simulink library "libturbines"  (R2025b)
settings: Solver=ode45  StartTime=0.0  StopTime=10.0  RelTol=1e-3  EnableMultiTasking=on
undefined symbols (not defined in the file): DiscIntNeverNeededParam, dt, faultOptions, noiseFlag
libraries: simulink x57, $bdroot x3
(part 4 of 5)

== system libturbines/Floating NREL5MW faulty/Controller/Region check ==
  Torque_dem : Inport
  w_gen : Inport  Port=2
  p_dem : Inport  Port=3
  pitch command : Inport  Port=4
  Demand limitation : RelationalOperator  Operator=<=  OutDataTypeStr=boolean  InputSameDT=off
  Divide : Product  Inputs=*/
  Enable Pitch control? : Logic  Operator=OR  Inputs=3  AllPortsSameDT=off  OutDataTypeStr=boolean
  Integer Delay : Delay  DelayLength=1
  Pitch actuator active last time? : simulink/Logic and Bit Operations/Compare To Constant  relop=>  const=wt.ctrl.torq.beta  OutDataTypeStr=uint8  ZeroCross=off
  Product : Product  RndMeth=Zero
  Region 3 speed? : simulink/Logic and Bit Operations/Compare To Constant  relop=>=  const=wt.ctrl.torq.r3  OutDataTypeStr=uint8  ZeroCross=off
  Switch Torque_ref : Switch  Threshold=1  SaturateOnIntegerOverflow=off  InputSameDT=off
  Torque_ref : Outport
  Enable pitch controller : Outport  Port=2
  wires:
  Divide/1 -> Switch Torque_ref/1
  Switch Torque_ref/1 -> Torque_ref/1
  Demand limitation/1 -> Enable Pitch control?/1
  p_dem/1 -> Divide/1, Demand limitation/1
  Torque_dem/1 -> Switch Torque_ref/3, Product/1
  Product/1 -> Demand limitation/2
  Enable Pitch control?/1 -> Switch Torque_ref/2, Enable pitch controller/1
  Integer Delay/1 -> Pitch actuator active last time?/1
  Region 3 speed?/1 -> Enable Pitch control?/2
  Pitch actuator active last time?/1 -> Enable Pitch control?/3
  w_gen/1 -> Product/2, Region 3 speed?/1, Divide/2
  pitch command/1 -> Integer Delay/1

== system libturbines/Floating NREL5MW faulty/Pitch Actuator/Pitch subsystems ==
  beta_ref [deg] : Inport
  Fault type 5 : Inport  Port=2
  Demux2 : Demux  Outputs=3
  Mux1 : Mux  Inputs=3
  Pitch system B1 : StateSpace  A=wt.pitch.ssA  B=wt.pitch.ssB  C=wt.pitch.ssC  D=wt.pitch.ssD  InitialCondition=0
  Pitch system B2 : StateSpace  A=wt.pitch.ssA  B=wt.pitch.ssB  C=wt.pitch.ssC  D=wt.pitch.ssD  InitialCondition=0
  Pitch system B3 : Subsystem
  beta [deg] : Outport
  wires:
  Pitch system B3/1(beta [deg]) -> Mux1/3
  Demux2/3 -> Pitch system B3/1(beta_ref [deg])
  Fault type 5/1 -> Pitch system B3/2(fault 5)
  beta_ref [deg]/1 -> Demux2/1
  Mux1/1 -> beta [deg]/1
  Pitch system B2/1 -> Mux1/2
  Pitch system B1/1 -> Mux1/1
  Demux2/1 -> Pitch system B1/1
  Demux2/2 -> Pitch system B2/1

== system libturbines/Floating NREL5MW faulty/Sensors sampling/generator encoder ==
  w_gen_in : Inport
  Sum : Sum  Inputs=-+|
  gen Integrator : Integrator  InitialCondition=wt.gen.ini
  gen sensor time constant : Gain  Gain=1/wt.meas.gentau
  w_gen_out : Outport
  wires:
  gen Integrator/1 -> w_gen_out/1, Sum/1
  Sum/1 -> gen sensor time constant/1
  gen sensor time constant/1 -> gen Integrator/1
  w_gen_in/1 -> Sum/2

== system libturbines/Floating NREL5MW faulty/Sensors sampling/rotor encoder ==
  w_rot_in : Inport
  Sum1 : Sum  Inputs=|+-
  gen Integrator1 : Integrator  InitialCondition=wt.rotor.ini
  gen sensor time constant1 : Gain  Gain=1/wt.meas.rottau
  w_rot_out : Outport
  wires:
  w_rot_in/1 -> Sum1/1
  gen Integrator1/1 -> w_rot_out/1, Sum1/2
  Sum1/1 -> gen sensor time constant1/1
  gen sensor time constant1/1 -> gen Integrator1/1

== system libturbines/Floating NREL5MW faulty/Tower deflection /Tower1 ==
  FT [Nm] : Inport
  Demux1 : Demux  Outputs=2
  Tower : StateSpace  A=A  B=B  C=C  D=D  InitialCondition=zeros(2,1)
  vnac [m/s] : Outport  InitialOutput=0
  F_tow [N] : Outport  Port=2  InitialOutput=0
  wires:
  Demux1/2 -> F_tow [N]/1
  FT [Nm]/1 -> Tower/1
  Demux1/1 -> vnac [m/s]/1
  Tower/1 -> Demux1/1

== system libturbines/Floating IEA15MW/Controller/Pitch controller/Blade 1 controller ==
  w_gen_diff : Inport
  P_dem : Inport  Port=2
  beta_meas [deg] : Inport  Port=3
  Discrete-Time Integrator : DiscreteIntegrator  SampleTime=wt.ctrl.Ts  LimitOutput=on  UpperSaturationLimit=wt.ctrl.pitch.ulim*pi/180  LowerSaturationLimit=wt.ctrl.pitch.llim  ICPrevOutput=DiscIntNeverNeededParam  ICPrevScaledInput=DiscIntNeverNeededParam
  Gain correction : Lookup2D  RowIndex=wt.ctrl.pitch.pwr  ColumnIndex=wt.ctrl.pitch.beta  Table=wt.ctrl.pitch.gs  LookUpMeth=Interpolation-Use End Values  SaturateOnIntegerOverflow=off  InputSameDT=off
  Integral gain : Gain  Gain=(1-0.999*noiseFlag)*wt.ctrl.pitch.Igain
  Integral schedule : Product  Inputs=*/  RndMeth=Zero
  Prop schedule : Product  Inputs=*/  RndMeth=Zero
  Proportional gain : Gain  Gain=(1-0.3*noiseFlag)*wt.ctrl.pitch.Pgain
  Rate Limiter : RateLimiter  RisingSlewLimit=wt.ctrl.pitch.ratelim  FallingSlewLimit=-wt.ctrl.pitch.ratelim  SampleTimeMode=inherited  InitialCondition=wt.ctrl.pitch.ini
  Saturation : Saturate  UpperLimit=wt.ctrl.pitch.ulim  LowerLimit=0
  Sum : Sum  Inputs=++|
  To degrees : Gain  Gain=180/pi
  beta_ref [deg] : Outport
  wires:
  Integral schedule/1 -> Discrete-Time Integrator/1
  Integral gain/1 -> Integral schedule/1
  Gain correction/1 -> Prop schedule/2, Integral schedule/2
  Sum/1 -> To degrees/1
  w_gen_diff/1 -> Integral gain/1, Proportional gain/1
  To degrees/1 -> Saturation/1
  Prop schedule/1 -> Sum/1
  Saturation/1 -> Rate Limiter/1
  Discrete-Time Integrator/1 -> Sum/2
  Proportional gain/1 -> Prop schedule/1
  beta_meas [deg]/1 -> Gain correction/2
  Rate Limiter/1 -> beta_ref [deg]/1
  P_dem/1 -> Gain correction/1

== system libturbines/Floating IEA15MW faulty/Aerodynamics/Blade 1/C_P & C_T tables ==
  beta : Inport
  lambda : Inport  Port=2
  "C_P table " : Lookup2D  RowIndex=wt.cp.beta  ColumnIndex=wt.cp.tsr  Table=wt.cp.table  LookUpMeth=Interpolation-Use End Values
  C_T table : Lookup2D  RowIndex=wt.ct.beta  ColumnIndex=wt.ct.tsr  Table=wt.ct.table  LookUpMeth=Interpolation-Use End Values
  C_T : Outport
  C_P : Outport  Port=2
  wires:
  lambda/1 -> "C_P table "/2, C_T table/2
  beta/1 -> "C_P table "/1, C_T table/1
  "C_P table "/1 -> C_P/1
  C_T table/1 -> C_T/1

== system libturbines/Floating IEA15MW faulty/Aerodynamics/Blade 2/C_P & C_T tables ==
  beta : Inport
  lambda : Inport  Port=2
  "C_P table " : Lookup2D  RowIndex=wt.cp.beta  ColumnIndex=wt.cp.tsr  Table=wt.cp.table  LookUpMeth=Interpolation-Use End Values
  C_T table : Lookup2D  RowIndex=wt.ct.beta  ColumnIndex=wt.ct.tsr  Table=wt.ct.table  LookUpMeth=Interpolation-Use End Values
  C_T : Outport
  C_P : Outport  Port=2
  wires:
  lambda/1 -> "C_P table "/2, C_T table/2
  beta/1 -> "C_P table "/1, C_T table/1
  "C_P table "/1 -> C_P/1
  C_T table/1 -> C_T/1

== system libturbines/Floating IEA15MW faulty/Aerodynamics/Blade 3/C_P & C_T tables ==
  beta : Inport
  lambda : Inport  Port=2
  "C_P table " : Lookup2D  RowIndex=wt.cp.beta  ColumnIndex=wt.cp.tsr  Table=wt.cp.table  LookUpMeth=Interpolation-Use End Values
  C_T table : Lookup2D  RowIndex=wt.ct.beta  ColumnIndex=wt.ct.tsr  Table=wt.ct.table  LookUpMeth=Interpolation-Use End Values
  C_T : Outport
  C_P : Outport  Port=2
  wires:
  lambda/1 -> "C_P table "/2, C_T table/2
  beta/1 -> "C_P table "/1, C_T table/1
  "C_P table "/1 -> C_P/1
  C_T table/1 -> C_T/1

== system libturbines/Floating IEA15MW faulty/Controller/Pitch controller/Blade 1 controller ==
  w_gen_diff : Inport
  P_dem : Inport  Port=2
  beta_meas [deg] : Inport  Port=3
  Discrete-Time Integrator : DiscreteIntegrator  SampleTime=wt.ctrl.Ts  LimitOutput=on  UpperSaturationLimit=wt.ctrl.pitch.ulim*pi/180  LowerSaturationLimit=wt.ctrl.pitch.llim  ICPrevOutput=DiscIntNeverNeededParam  ICPrevScaledInput=DiscIntNeverNeededParam
  Gain correction : Lookup2D  RowIndex=wt.ctrl.pitch.pwr  ColumnIndex=wt.ctrl.pitch.beta  Table=wt.ctrl.pitch.gs  LookUpMeth=Interpolation-Use End Values  SaturateOnIntegerOverflow=off  InputSameDT=off
  Integral gain : Gain  Gain=(1-0.999*noiseFlag)*wt.ctrl.pitch.Igain
  Integral schedule : Product  Inputs=*/  RndMeth=Zero
  Prop schedule : Product  Inputs=*/  RndMeth=Zero
  Proportional gain : Gain  Gain=(1-0.3*noiseFlag)*wt.ctrl.pitch.Pgain
  Rate Limiter : RateLimiter  RisingSlewLimit=wt.ctrl.pitch.ratelim  FallingSlewLimit=-wt.ctrl.pitch.ratelim  SampleTimeMode=inherited  InitialCondition=wt.ctrl.pitch.ini
  Saturation : Saturate  UpperLimit=wt.ctrl.pitch.ulim  LowerLimit=0
  Sum : Sum  Inputs=++|
  To degrees : Gain  Gain=180/pi
  beta_ref [deg] : Outport
  wires:
  P_dem/1 -> Gain correction/1
  Rate Limiter/1 -> beta_ref [deg]/1
  beta_meas [deg]/1 -> Gain correction/2
  Proportional gain/1 -> Prop schedule/1
  Discrete-Time Integrator/1 -> Sum/2
  Saturation/1 -> Rate Limiter/1
  Prop schedule/1 -> Sum/1
  To degrees/1 -> Saturation/1
  w_gen_diff/1 -> Integral gain/1, Proportional gain/1
  Sum/1 -> To degrees/1
  Gain correction/1 -> Integral schedule/2, Prop schedule/2
  Integral gain/1 -> Integral schedule/1
  Integral schedule/1 -> Discrete-Time Integrator/1

== system libturbines/Floating IEA15MW faulty/Controller/Pitch controller/Blade 2 controller ==
  w_gen_diff : Inport
  P_dem : Inport  Port=2
  beta_meas [deg] : Inport  Port=3
  Discrete-Time Integrator : DiscreteIntegrator  SampleTime=wt.ctrl.Ts  LimitOutput=on  UpperSaturationLimit=wt.ctrl.pitch.ulim*pi/180  LowerSaturationLimit=wt.ctrl.pitch.llim  ICPrevOutput=DiscIntNeverNeededParam  ICPrevScaledInput=DiscIntNeverNeededParam
  Gain correction : Lookup2D  RowIndex=wt.ctrl.pitch.pwr  ColumnIndex=wt.ctrl.pitch.beta  Table=wt.ctrl.pitch.gs  LookUpMeth=Interpolation-Use End Values  SaturateOnIntegerOverflow=off  InputSameDT=off
  Integral gain : Gain  Gain=(1-0.999*noiseFlag)*wt.ctrl.pitch.Igain
  Integral schedule : Product  Inputs=*/  RndMeth=Zero
  Prop schedule : Product  Inputs=*/  RndMeth=Zero
  Proportional gain : Gain  Gain=(1-0.3*noiseFlag)*wt.ctrl.pitch.Pgain
  Rate Limiter : RateLimiter  RisingSlewLimit=wt.ctrl.pitch.ratelim  FallingSlewLimit=-wt.ctrl.pitch.ratelim  SampleTimeMode=inherited  InitialCondition=wt.ctrl.pitch.ini
  Saturation : Saturate  UpperLimit=wt.ctrl.pitch.ulim  LowerLimit=0
  Sum : Sum  Inputs=++|
  To degrees : Gain  Gain=180/pi
  beta_ref [deg] : Outport
  wires:
  Integral schedule/1 -> Discrete-Time Integrator/1
  Integral gain/1 -> Integral schedule/1
  Gain correction/1 -> Prop schedule/2, Integral schedule/2
  Sum/1 -> To degrees/1
  w_gen_diff/1 -> Proportional gain/1, Integral gain/1
  To degrees/1 -> Saturation/1
  Prop schedule/1 -> Sum/1
  Saturation/1 -> Rate Limiter/1
  Discrete-Time Integrator/1 -> Sum/2
  Proportional gain/1 -> Prop schedule/1
  beta_meas [deg]/1 -> Gain correction/2
  Rate Limiter/1 -> beta_ref [deg]/1
  P_dem/1 -> Gain correction/1

== system libturbines/Floating IEA15MW faulty/Controller/Pitch controller/Blade 3 controller ==
  w_gen_diff : Inport
  P_dem : Inport  Port=2
  beta_meas [deg] : Inport  Port=3
  Discrete-Time Integrator : DiscreteIntegrator  SampleTime=wt.ctrl.Ts  LimitOutput=on  UpperSaturationLimit=wt.ctrl.pitch.ulim*pi/180  LowerSaturationLimit=wt.ctrl.pitch.llim  ICPrevOutput=DiscIntNeverNeededParam  ICPrevScaledInput=DiscIntNeverNeededParam
  Gain correction : Lookup2D  RowIndex=wt.ctrl.pitch.pwr  ColumnIndex=wt.ctrl.pitch.beta  Table=wt.ctrl.pitch.gs  LookUpMeth=Interpolation-Use End Values  SaturateOnIntegerOverflow=off  InputSameDT=off
  Integral gain : Gain  Gain=(1-0.999*noiseFlag)*wt.ctrl.pitch.Igain
  Integral schedule : Product  Inputs=*/  RndMeth=Zero
  Prop schedule : Product  Inputs=*/  RndMeth=Zero
  Proportional gain : Gain  Gain=(1-0.3*noiseFlag)*wt.ctrl.pitch.Pgain
  Rate Limiter : RateLimiter  RisingSlewLimit=wt.ctrl.pitch.ratelim  FallingSlewLimit=-wt.ctrl.pitch.ratelim  SampleTimeMode=inherited  InitialCondition=wt.ctrl.pitch.ini
  Saturation : Saturate  UpperLimit=wt.ctrl.pitch.ulim  LowerLimit=0
  Sum : Sum  Inputs=++|
  To degrees : Gain  Gain=180/pi
  beta_ref [deg] : Outport
  wires:
  P_dem/1 -> Gain correction/1
  Rate Limiter/1 -> beta_ref [deg]/1
  beta_meas [deg]/1 -> Gain correction/2
  Proportional gain/1 -> Prop schedule/1
  Discrete-Time Integrator/1 -> Sum/2
  Saturation/1 -> Rate Limiter/1
  Prop schedule/1 -> Sum/1
  To degrees/1 -> Saturation/1
  w_gen_diff/1 -> Integral gain/1, Proportional gain/1
  Sum/1 -> To degrees/1
  Gain correction/1 -> Integral schedule/2, Prop schedule/2
  Integral gain/1 -> Integral schedule/1
  Integral schedule/1 -> Discrete-Time Integrator/1

== system libturbines/Floating IEA15MW faulty/Pitch Actuator/Pitch subsystems/Pitch system B3 ==
  beta_ref [deg] : Inport
  fault 5 : Inport  Port=2
  Compare To Constant : simulink/Logic and Bit Operations/Compare To Constant  relop===  const=5  OutDataTypeStr=boolean
  Constant : Constant  Value=wt.pitch.omega
  Constant1 : Constant  Value=wt.pitch.damp
  Constant2 : Constant
  Constant3 : Constant  Value=faultOptions.pitchNatFreq
  Constant4 : Constant  Value=faultOptions.pitchDamp
  Demux1 : Demux  Outputs=2
  Gain2 : Gain  Gain=2
  Integrator : Integrator
  Integrator1 : Integrator
  Product{1..3,5} (4 alike) : Product
  Signal Specification : SignalSpecification  OutDataTypeStr=double  Dimensions=1
  Square : Math  Operator=square
  Sum : Sum  Inputs=-+-
  Sum1 : Sum  Inputs=|+-
  Switch1 : Switch  Criteria=u2 ~= 0  SaturateOnIntegerOverflow=off  InputSameDT=off
  mux1 : Mux  Inputs=2
  mux2 : Mux  Inputs=2
  beta [deg] : Outport
  wires:
  Sum1/1 -> Switch1/2
  Product1/1 -> Sum/2
  Product3/1 -> Sum/1
  Constant/1 -> mux1/1
  Gain2/1 -> Product2/2
  Integrator1/1 -> Signal Specification/1, Product3/2
  Demux1/2 -> Product5/2
  Integrator/1 -> Product2/1, Integrator1/1
  Compare To Constant/1 -> Sum1/1
  Demux1/1 -> Product5/1, Square/1
  fault 5/1 -> Compare To Constant/1
  Constant2/1 -> Sum1/2
  Signal Specification/1 -> beta [deg]/1
  mux2/1 -> Switch1/3
  Sum/1 -> Integrator/1
  Square/1 -> Product3/1, Product1/2
  beta_ref [deg]/1 -> Product1/1
  Constant4/1 -> mux2/2
  mux1/1 -> Switch1/1
  Constant1/1 -> mux1/2
  Constant3/1 -> mux2/1
  Product5/1 -> Gain2/1
  Switch1/1 -> Demux1/1
  Product2/1 -> Sum/3

== system libturbines/Floating IEA3.4MW/Controller/Pitch controller/Blade 1 controller ==
  w_gen_diff : Inport
  P_dem : Inport  Port=2
  beta_meas [deg] : Inport  Port=3
  Discrete-Time Integrator : DiscreteIntegrator  SampleTime=wt.ctrl.Ts  LimitOutput=on  UpperSaturationLimit=wt.ctrl.pitch.ulim*pi/180  LowerSaturationLimit=wt.ctrl.pitch.llim  ICPrevOutput=DiscIntNeverNeededParam  ICPrevScaledInput=DiscIntNeverNeededParam
  Gain correction : Lookup2D  RowIndex=wt.ctrl.pitch.pwr  ColumnIndex=wt.ctrl.pitch.beta  Table=wt.ctrl.pitch.gs  LookUpMeth=Interpolation-Use End Values  SaturateOnIntegerOverflow=off  InputSameDT=off
  Integral gain : Gain  Gain=(1-0.999*noiseFlag)*wt.ctrl.pitch.Igain
  Integral schedule : Product  Inputs=*/  RndMeth=Zero
  Prop schedule : Product  Inputs=*/  RndMeth=Zero
  Proportional gain : Gain  Gain=(1-0.3*noiseFlag)*wt.ctrl.pitch.Pgain
  Rate Limiter : RateLimiter  RisingSlewLimit=wt.ctrl.pitch.ratelim  FallingSlewLimit=-wt.ctrl.pitch.ratelim  SampleTimeMode=inherited  InitialCondition=wt.ctrl.pitch.ini
  Saturation : Saturate  UpperLimit=wt.ctrl.pitch.ulim  LowerLimit=0
  Sum : Sum  Inputs=++|
  To degrees : Gain  Gain=180/pi
  beta_ref [deg] : Outport
  wires:
  Integral schedule/1 -> Discrete-Time Integrator/1
  Integral gain/1 -> Integral schedule/1
  Gain correction/1 -> Prop schedule/2, Integral schedule/2
  Sum/1 -> To degrees/1
  w_gen_diff/1 -> Integral gain/1, Proportional gain/1
  To degrees/1 -> Saturation/1
  Prop schedule/1 -> Sum/1
  Saturation/1 -> Rate Limiter/1
  Discrete-Time Integrator/1 -> Sum/2
  Proportional gain/1 -> Prop schedule/1
  beta_meas [deg]/1 -> Gain correction/2
  Rate Limiter/1 -> beta_ref [deg]/1
  P_dem/1 -> Gain correction/1

== system libturbines/Floating IEA3.4MW faulty/Aerodynamics/Blade 1/C_P & C_T tables ==
  beta : Inport
  lambda : Inport  Port=2
  "C_P table " : Lookup2D  RowIndex=wt.cp.beta  ColumnIndex=wt.cp.tsr  Table=wt.cp.table  LookUpMeth=Interpolation-Use End Values
  C_T table : Lookup2D  RowIndex=wt.ct.beta  ColumnIndex=wt.ct.tsr  Table=wt.ct.table  LookUpMeth=Interpolation-Use End Values
  C_T : Outport
  C_P : Outport  Port=2
  wires:
  lambda/1 -> "C_P table "/2, C_T table/2
  beta/1 -> "C_P table "/1, C_T table/1
  "C_P table "/1 -> C_P/1
  C_T table/1 -> C_T/1

== system libturbines/Floating IEA3.4MW faulty/Aerodynamics/Blade 2/C_P & C_T tables ==
  beta : Inport
  lambda : Inport  Port=2
  "C_P table " : Lookup2D  RowIndex=wt.cp.beta  ColumnIndex=wt.cp.tsr  Table=wt.cp.table  LookUpMeth=Interpolation-Use End Values
  C_T table : Lookup2D  RowIndex=wt.ct.beta  ColumnIndex=wt.ct.tsr  Table=wt.ct.table  LookUpMeth=Interpolation-Use End Values
  C_T : Outport
  C_P : Outport  Port=2
  wires:
  lambda/1 -> "C_P table "/2, C_T table/2
  beta/1 -> "C_P table "/1, C_T table/1
  "C_P table "/1 -> C_P/1
  C_T table/1 -> C_T/1

== system libturbines/Floating IEA3.4MW faulty/Aerodynamics/Blade 3/C_P & C_T tables ==
  beta : Inport
  lambda : Inport  Port=2
  "C_P table " : Lookup2D  RowIndex=wt.cp.beta  ColumnIndex=wt.cp.tsr  Table=wt.cp.table  LookUpMeth=Interpolation-Use End Values
  C_T table : Lookup2D  RowIndex=wt.ct.beta  ColumnIndex=wt.ct.tsr  Table=wt.ct.table  LookUpMeth=Interpolation-Use End Values
  C_T : Outport
  C_P : Outport  Port=2
  wires:
  lambda/1 -> "C_P table "/2, C_T table/2
  beta/1 -> "C_P table "/1, C_T table/1
  "C_P table "/1 -> C_P/1
  C_T table/1 -> C_T/1

== system libturbines/Floating IEA3.4MW faulty/Controller/Pitch controller/Blade 1 controller ==
  w_gen_diff : Inport
  P_dem : Inport  Port=2
  beta_meas [deg] : Inport  Port=3
  Discrete-Time Integrator : DiscreteIntegrator  SampleTime=wt.ctrl.Ts  LimitOutput=on  UpperSaturationLimit=wt.ctrl.pitch.ulim*pi/180  LowerSaturationLimit=wt.ctrl.pitch.llim  ICPrevOutput=DiscIntNeverNeededParam  ICPrevScaledInput=DiscIntNeverNeededParam
  Gain correction : Lookup2D  RowIndex=wt.ctrl.pitch.pwr  ColumnIndex=wt.ctrl.pitch.beta  Table=wt.ctrl.pitch.gs  LookUpMeth=Interpolation-Use End Values  SaturateOnIntegerOverflow=off  InputSameDT=off
  Integral gain : Gain  Gain=(1-0.999*noiseFlag)*wt.ctrl.pitch.Igain
  Integral schedule : Product  Inputs=*/  RndMeth=Zero
  Prop schedule : Product  Inputs=*/  RndMeth=Zero
  Proportional gain : Gain  Gain=(1-0.3*noiseFlag)*wt.ctrl.pitch.Pgain
  Rate Limiter : RateLimiter  RisingSlewLimit=wt.ctrl.pitch.ratelim  FallingSlewLimit=-wt.ctrl.pitch.ratelim  SampleTimeMode=inherited  InitialCondition=wt.ctrl.pitch.ini
  Saturation : Saturate  UpperLimit=wt.ctrl.pitch.ulim  LowerLimit=0
  Sum : Sum  Inputs=++|
  To degrees : Gain  Gain=180/pi
  beta_ref [deg] : Outport
  wires:
  P_dem/1 -> Gain correction/1
  Rate Limiter/1 -> beta_ref [deg]/1
  beta_meas [deg]/1 -> Gain correction/2
  Proportional gain/1 -> Prop schedule/1
  Discrete-Time Integrator/1 -> Sum/2
  Saturation/1 -> Rate Limiter/1
  Prop schedule/1 -> Sum/1
  To degrees/1 -> Saturation/1
  w_gen_diff/1 -> Integral gain/1, Proportional gain/1
  Sum/1 -> To degrees/1
  Gain correction/1 -> Integral schedule/2, Prop schedule/2
  Integral gain/1 -> Integral schedule/1
  Integral schedule/1 -> Discrete-Time Integrator/1

== system libturbines/Floating IEA3.4MW faulty/Controller/Pitch controller/Blade 2 controller ==
  w_gen_diff : Inport
  P_dem : Inport  Port=2
  beta_meas [deg] : Inport  Port=3
  Discrete-Time Integrator : DiscreteIntegrator  SampleTime=wt.ctrl.Ts  LimitOutput=on  UpperSaturationLimit=wt.ctrl.pitch.ulim*pi/180  LowerSaturationLimit=wt.ctrl.pitch.llim  ICPrevOutput=DiscIntNeverNeededParam  ICPrevScaledInput=DiscIntNeverNeededParam
  Gain correction : Lookup2D  RowIndex=wt.ctrl.pitch.pwr  ColumnIndex=wt.ctrl.pitch.beta  Table=wt.ctrl.pitch.gs  LookUpMeth=Interpolation-Use End Values  SaturateOnIntegerOverflow=off  InputSameDT=off
  Integral gain : Gain  Gain=(1-0.999*noiseFlag)*wt.ctrl.pitch.Igain
  Integral schedule : Product  Inputs=*/  RndMeth=Zero
  Prop schedule : Product  Inputs=*/  RndMeth=Zero
  Proportional gain : Gain  Gain=(1-0.3*noiseFlag)*wt.ctrl.pitch.Pgain
  Rate Limiter : RateLimiter  RisingSlewLimit=wt.ctrl.pitch.ratelim  FallingSlewLimit=-wt.ctrl.pitch.ratelim  SampleTimeMode=inherited  InitialCondition=wt.ctrl.pitch.ini
  Saturation : Saturate  UpperLimit=wt.ctrl.pitch.ulim  LowerLimit=0
  Sum : Sum  Inputs=++|
  To degrees : Gain  Gain=180/pi
  beta_ref [deg] : Outport
  wires:
  Integral schedule/1 -> Discrete-Time Integrator/1
  Integral gain/1 -> Integral schedule/1
  Gain correction/1 -> Prop schedule/2, Integral schedule/2
  Sum/1 -> To degrees/1
  w_gen_diff/1 -> Proportional gain/1, Integral gain/1
  To degrees/1 -> Saturation/1
  Prop schedule/1 -> Sum/1
  Saturation/1 -> Rate Limiter/1
  Discrete-Time Integrator/1 -> Sum/2
  Proportional gain/1 -> Prop schedule/1
  beta_meas [deg]/1 -> Gain correction/2
  Rate Limiter/1 -> beta_ref [deg]/1
  P_dem/1 -> Gain correction/1

== system libturbines/Floating IEA3.4MW faulty/Controller/Pitch controller/Blade 3 controller ==
  w_gen_diff : Inport
  P_dem : Inport  Port=2
  beta_meas [deg] : Inport  Port=3
  Discrete-Time Integrator : DiscreteIntegrator  SampleTime=wt.ctrl.Ts  LimitOutput=on  UpperSaturationLimit=wt.ctrl.pitch.ulim*pi/180  LowerSaturationLimit=wt.ctrl.pitch.llim  ICPrevOutput=DiscIntNeverNeededParam  ICPrevScaledInput=DiscIntNeverNeededParam
  Gain correction : Lookup2D  RowIndex=wt.ctrl.pitch.pwr  ColumnIndex=wt.ctrl.pitch.beta  Table=wt.ctrl.pitch.gs  LookUpMeth=Interpolation-Use End Values  SaturateOnIntegerOverflow=off  InputSameDT=off
  Integral gain : Gain  Gain=(1-0.999*noiseFlag)*wt.ctrl.pitch.Igain
  Integral schedule : Product  Inputs=*/  RndMeth=Zero
  Prop schedule : Product  Inputs=*/  RndMeth=Zero
  Proportional gain : Gain  Gain=(1-0.3*noiseFlag)*wt.ctrl.pitch.Pgain
  Rate Limiter : RateLimiter  RisingSlewLimit=wt.ctrl.pitch.ratelim  FallingSlewLimit=-wt.ctrl.pitch.ratelim  SampleTimeMode=inherited  InitialCondition=wt.ctrl.pitch.ini
  Saturation : Saturate  UpperLimit=wt.ctrl.pitch.ulim  LowerLimit=0
  Sum : Sum  Inputs=++|
  To degrees : Gain  Gain=180/pi
  beta_ref [deg] : Outport
  wires:
  P_dem/1 -> Gain correction/1
  Rate Limiter/1 -> beta_ref [deg]/1
  beta_meas [deg]/1 -> Gain correction/2
  Proportional gain/1 -> Prop schedule/1
  Discrete-Time Integrator/1 -> Sum/2
  Saturation/1 -> Rate Limiter/1
  Prop schedule/1 -> Sum/1
  To degrees/1 -> Saturation/1
  w_gen_diff/1 -> Integral gain/1, Proportional gain/1
  Sum/1 -> To degrees/1
  Gain correction/1 -> Integral schedule/2, Prop schedule/2
  Integral gain/1 -> Integral schedule/1
  Integral schedule/1 -> Discrete-Time Integrator/1

== system libturbines/Floating IEA3.4MW faulty/Pitch Actuator/Pitch subsystems/Pitch system B3 ==
  beta_ref [deg] : Inport
  fault 5 : Inport  Port=2
  Compare To Constant : simulink/Logic and Bit Operations/Compare To Constant  relop===  const=5  OutDataTypeStr=boolean
  Constant : Constant  Value=wt.pitch.omega
  Constant1 : Constant  Value=wt.pitch.damp
  Constant2 : Constant
  Constant3 : Constant  Value=faultOptions.pitchNatFreq
  Constant4 : Constant  Value=faultOptions.pitchDamp
  Demux1 : Demux  Outputs=2
  Gain2 : Gain  Gain=2
  Integrator : Integrator
  Integrator1 : Integrator
  Product{1..3,5} (4 alike) : Product
  Signal Specification : SignalSpecification  OutDataTypeStr=double  Dimensions=1
  Square : Math  Operator=square
  Sum : Sum  Inputs=-+-
  Sum1 : Sum  Inputs=|+-
  Switch1 : Switch  Criteria=u2 ~= 0  SaturateOnIntegerOverflow=off  InputSameDT=off
  mux1 : Mux  Inputs=2
  mux2 : Mux  Inputs=2
  beta [deg] : Outport
  wires:
  Sum1/1 -> Switch1/2
  Product1/1 -> Sum/2
  Product3/1 -> Sum/1
  Constant/1 -> mux1/1
  Gain2/1 -> Product2/2
  Integrator1/1 -> Signal Specification/1, Product3/2
  Demux1/2 -> Product5/2
  Integrator/1 -> Product2/1, Integrator1/1
  Compare To Constant/1 -> Sum1/1
  Demux1/1 -> Product5/1, Square/1
  fault 5/1 -> Compare To Constant/1
  Constant2/1 -> Sum1/2
  Signal Specification/1 -> beta [deg]/1
  mux2/1 -> Switch1/3
  Sum/1 -> Integrator/1
  Square/1 -> Product3/1, Product1/2
  beta_ref [deg]/1 -> Product1/1
  Constant4/1 -> mux2/2
  mux1/1 -> Switch1/1
  Constant1/1 -> mux1/2
  Constant3/1 -> mux2/1
  Product5/1 -> Gain2/1
  Switch1/1 -> Demux1/1
  Product2/1 -> Sum/3

== system libturbines/Floating NREL5MW/Controller/Pitch controller/Blade 1 controller ==
  w_gen_diff : Inport
  P_dem : Inport  Port=2
  beta_meas [deg] : Inport  Port=3
  Discrete-Time Integrator : DiscreteIntegrator  SampleTime=wt.ctrl.Ts  LimitOutput=on  UpperSaturationLimit=wt.ctrl.pitch.ulim*pi/180  LowerSaturationLimit=wt.ctrl.pitch.llim  ICPrevOutput=DiscIntNeverNeededParam  ICPrevScaledInput=DiscIntNeverNeededParam
  Gain correction : Lookup2D  RowIndex=wt.ctrl.pitch.pwr  ColumnIndex=wt.ctrl.pitch.beta  Table=wt.ctrl.pitch.gs  LookUpMeth=Interpolation-Use End Values  SaturateOnIntegerOverflow=off  InputSameDT=off
  Integral gain : Gain  Gain=(1-0.999*noiseFlag)*wt.ctrl.pitch.Igain
  Integral schedule : Product  Inputs=*/  RndMeth=Zero
  Prop schedule : Product  Inputs=*/  RndMeth=Zero
  Proportional gain : Gain  Gain=(1-0.3*noiseFlag)*wt.ctrl.pitch.Pgain
  Rate Limiter : RateLimiter  RisingSlewLimit=wt.ctrl.pitch.ratelim  FallingSlewLimit=-wt.ctrl.pitch.ratelim  SampleTimeMode=inherited  InitialCondition=wt.ctrl.pitch.ini
  Saturation : Saturate  UpperLimit=wt.ctrl.pitch.ulim  LowerLimit=0
  Sum : Sum  Inputs=++|
  To degrees : Gain  Gain=180/pi
  beta_ref [deg] : Outport
  wires:
  P_dem/1 -> Gain correction/1
  Rate Limiter/1 -> beta_ref [deg]/1
  beta_meas [deg]/1 -> Gain correction/2
  Proportional gain/1 -> Prop schedule/1
  Discrete-Time Integrator/1 -> Sum/2
  Saturation/1 -> Rate Limiter/1
  Prop schedule/1 -> Sum/1
  To degrees/1 -> Saturation/1
  w_gen_diff/1 -> Proportional gain/1, Integral gain/1
  Sum/1 -> To degrees/1
  Gain correction/1 -> Integral schedule/2, Prop schedule/2
  Integral gain/1 -> Integral schedule/1
  Integral schedule/1 -> Discrete-Time Integrator/1

== system libturbines/Floating NREL5MW faulty/Aerodynamics/Blade 1/C_P & C_T tables ==
  beta : Inport
  lambda : Inport  Port=2
  "C_P table " : Lookup2D  RowIndex=wt.cp.beta  ColumnIndex=wt.cp.tsr  Table=wt.cp.table  LookUpMeth=Interpolation-Use End Values
  C_T table : Lookup2D  RowIndex=wt.ct.beta  ColumnIndex=wt.ct.tsr  Table=wt.ct.table  LookUpMeth=Interpolation-Use End Values
  C_T : Outport
  C_P : Outport  Port=2
  wires:
  C_T table/1 -> C_T/1
  "C_P table "/1 -> C_P/1
  beta/1 -> C_T table/1, "C_P table "/1
  lambda/1 -> C_T table/2, "C_P table "/2

== system libturbines/Floating NREL5MW faulty/Aerodynamics/Blade 2/C_P & C_T tables ==
  beta : Inport
  lambda : Inport  Port=2
  "C_P table " : Lookup2D  RowIndex=wt.cp.beta  ColumnIndex=wt.cp.tsr  Table=wt.cp.table  LookUpMeth=Interpolation-Use End Values
  C_T table : Lookup2D  RowIndex=wt.ct.beta  ColumnIndex=wt.ct.tsr  Table=wt.ct.table  LookUpMeth=Interpolation-Use End Values
  C_T : Outport
  C_P : Outport  Port=2
  wires:
  C_T table/1 -> C_T/1
  "C_P table "/1 -> C_P/1
  beta/1 -> C_T table/1, "C_P table "/1
  lambda/1 -> C_T table/2, "C_P table "/2

== system libturbines/Floating NREL5MW faulty/Aerodynamics/Blade 3/C_P & C_T tables ==
  beta : Inport
  lambda : Inport  Port=2
  "C_P table " : Lookup2D  RowIndex=wt.cp.beta  ColumnIndex=wt.cp.tsr  Table=wt.cp.table  LookUpMeth=Interpolation-Use End Values
  C_T table : Lookup2D  RowIndex=wt.ct.beta  ColumnIndex=wt.ct.tsr  Table=wt.ct.table  LookUpMeth=Interpolation-Use End Values
  C_T : Outport
  C_P : Outport  Port=2
  wires:
  C_T table/1 -> C_T/1
  "C_P table "/1 -> C_P/1
  beta/1 -> C_T table/1, "C_P table "/1
  lambda/1 -> C_T table/2, "C_P table "/2

== system libturbines/Floating NREL5MW faulty/Controller/Pitch controller/Blade 1 controller ==
  w_gen_diff : Inport
  P_dem : Inport  Port=2
  beta_meas [deg] : Inport  Port=3
  Discrete-Time Integrator : DiscreteIntegrator  SampleTime=wt.ctrl.Ts  LimitOutput=on  UpperSaturationLimit=wt.ctrl.pitch.ulim*pi/180  LowerSaturationLimit=wt.ctrl.pitch.llim  ICPrevOutput=DiscIntNeverNeededParam  ICPrevScaledInput=DiscIntNeverNeededParam
  Gain correction : Lookup2D  RowIndex=wt.ctrl.pitch.pwr  ColumnIndex=wt.ctrl.pitch.beta  Table=wt.ctrl.pitch.gs  LookUpMeth=Interpolation-Use End Values  SaturateOnIntegerOverflow=off  InputSameDT=off
  Integral gain : Gain  Gain=(1-0.999*noiseFlag)*wt.ctrl.pitch.Igain
  Integral schedule : Product  Inputs=*/  RndMeth=Zero
  Prop schedule : Product  Inputs=*/  RndMeth=Zero
  Proportional gain : Gain  Gain=(1-0.3*noiseFlag)*wt.ctrl.pitch.Pgain
  Rate Limiter : RateLimiter  RisingSlewLimit=wt.ctrl.pitch.ratelim  FallingSlewLimit=-wt.ctrl.pitch.ratelim  SampleTimeMode=inherited  InitialCondition=wt.ctrl.pitch.ini
  Saturation : Saturate  UpperLimit=wt.ctrl.pitch.ulim  LowerLimit=0
  Sum : Sum  Inputs=++|
  To degrees : Gain  Gain=180/pi
  beta_ref [deg] : Outport
  wires:
  Integral schedule/1 -> Discrete-Time Integrator/1
  Integral gain/1 -> Integral schedule/1
  Gain correction/1 -> Prop schedule/2, Integral schedule/2
  Sum/1 -> To degrees/1
  w_gen_diff/1 -> Proportional gain/1, Integral gain/1
  To degrees/1 -> Saturation/1
  Prop schedule/1 -> Sum/1
  Saturation/1 -> Rate Limiter/1
  Discrete-Time Integrator/1 -> Sum/2
  Proportional gain/1 -> Prop schedule/1
  beta_meas [deg]/1 -> Gain correction/2
  Rate Limiter/1 -> beta_ref [deg]/1
  P_dem/1 -> Gain correction/1

== system libturbines/Floating NREL5MW faulty/Controller/Pitch controller/Blade 2 controller ==
  w_gen_diff : Inport
  P_dem : Inport  Port=2
  beta_meas [deg] : Inport  Port=3
  Discrete-Time Integrator : DiscreteIntegrator  SampleTime=wt.ctrl.Ts  LimitOutput=on  UpperSaturationLimit=wt.ctrl.pitch.ulim*pi/180  LowerSaturationLimit=wt.ctrl.pitch.llim  ICPrevOutput=DiscIntNeverNeededParam  ICPrevScaledInput=DiscIntNeverNeededParam
  Gain correction : Lookup2D  RowIndex=wt.ctrl.pitch.pwr  ColumnIndex=wt.ctrl.pitch.beta  Table=wt.ctrl.pitch.gs  LookUpMeth=Interpolation-Use End Values  SaturateOnIntegerOverflow=off  InputSameDT=off
  Integral gain : Gain  Gain=(1-0.999*noiseFlag)*wt.ctrl.pitch.Igain
  Integral schedule : Product  Inputs=*/  RndMeth=Zero
  Prop schedule : Product  Inputs=*/  RndMeth=Zero
  Proportional gain : Gain  Gain=(1-0.3*noiseFlag)*wt.ctrl.pitch.Pgain
  Rate Limiter : RateLimiter  RisingSlewLimit=wt.ctrl.pitch.ratelim  FallingSlewLimit=-wt.ctrl.pitch.ratelim  SampleTimeMode=inherited  InitialCondition=wt.ctrl.pitch.ini
  Saturation : Saturate  UpperLimit=wt.ctrl.pitch.ulim  LowerLimit=0
  Sum : Sum  Inputs=++|
  To degrees : Gain  Gain=180/pi
  beta_ref [deg] : Outport
  wires:
  P_dem/1 -> Gain correction/1
  Rate Limiter/1 -> beta_ref [deg]/1
  beta_meas [deg]/1 -> Gain correction/2
  Proportional gain/1 -> Prop schedule/1
  Discrete-Time Integrator/1 -> Sum/2
  Saturation/1 -> Rate Limiter/1
  Prop schedule/1 -> Sum/1
  To degrees/1 -> Saturation/1
  w_gen_diff/1 -> Integral gain/1, Proportional gain/1
  Sum/1 -> To degrees/1
  Gain correction/1 -> Integral schedule/2, Prop schedule/2
  Integral gain/1 -> Integral schedule/1
  Integral schedule/1 -> Discrete-Time Integrator/1

== system libturbines/Floating NREL5MW faulty/Controller/Pitch controller/Blade 3 controller ==
  w_gen_diff : Inport
  P_dem : Inport  Port=2
  beta_meas [deg] : Inport  Port=3
  Discrete-Time Integrator : DiscreteIntegrator  SampleTime=wt.ctrl.Ts  LimitOutput=on  UpperSaturationLimit=wt.ctrl.pitch.ulim*pi/180  LowerSaturationLimit=wt.ctrl.pitch.llim  ICPrevOutput=DiscIntNeverNeededParam  ICPrevScaledInput=DiscIntNeverNeededParam
  Gain correction : Lookup2D  RowIndex=wt.ctrl.pitch.pwr  ColumnIndex=wt.ctrl.pitch.beta  Table=wt.ctrl.pitch.gs  LookUpMeth=Interpolation-Use End Values  SaturateOnIntegerOverflow=off  InputSameDT=off
  Integral gain : Gain  Gain=(1-0.999*noiseFlag)*wt.ctrl.pitch.Igain
  Integral schedule : Product  Inputs=*/  RndMeth=Zero
  Prop schedule : Product  Inputs=*/  RndMeth=Zero
  Proportional gain : Gain  Gain=(1-0.3*noiseFlag)*wt.ctrl.pitch.Pgain
  Rate Limiter : RateLimiter  RisingSlewLimit=wt.ctrl.pitch.ratelim  FallingSlewLimit=-wt.ctrl.pitch.ratelim  SampleTimeMode=inherited  InitialCondition=wt.ctrl.pitch.ini
  Saturation : Saturate  UpperLimit=wt.ctrl.pitch.ulim  LowerLimit=0
  Sum : Sum  Inputs=++|
  To degrees : Gain  Gain=180/pi
  beta_ref [deg] : Outport
  wires:
  Integral schedule/1 -> Discrete-Time Integrator/1
  Integral gain/1 -> Integral schedule/1
  Gain correction/1 -> Prop schedule/2, Integral schedule/2
  Sum/1 -> To degrees/1
  w_gen_diff/1 -> Proportional gain/1, Integral gain/1
  To degrees/1 -> Saturation/1
  Prop schedule/1 -> Sum/1
  Saturation/1 -> Rate Limiter/1
  Discrete-Time Integrator/1 -> Sum/2
  Proportional gain/1 -> Prop schedule/1
  beta_meas [deg]/1 -> Gain correction/2
  Rate Limiter/1 -> beta_ref [deg]/1
  P_dem/1 -> Gain correction/1

== system libturbines/Floating NREL5MW faulty/Pitch Actuator/Pitch subsystems/Pitch system B3 ==
  beta_ref [deg] : Inport
  fault 5 : Inport  Port=2
  Compare To Constant : simulink/Logic and Bit Operations/Compare To Constant  relop===  const=5  OutDataTypeStr=boolean
  Constant : Constant  Value=wt.pitch.omega
  Constant1 : Constant  Value=wt.pitch.damp
  Constant2 : Constant
  Constant3 : Constant  Value=faultOptions.pitchNatFreq
  Constant4 : Constant  Value=faultOptions.pitchDamp
  Demux1 : Demux  Outputs=2
  Gain2 : Gain  Gain=2
  Integrator : Integrator
  Integrator1 : Integrator
  Product{1..3,5} (4 alike) : Product
  Signal Specification : SignalSpecification  OutDataTypeStr=double  Dimensions=1
  Square : Math  Operator=square
  Sum : Sum  Inputs=-+-
  Sum1 : Sum  Inputs=|+-
  Switch1 : Switch  Criteria=u2 ~= 0  SaturateOnIntegerOverflow=off  InputSameDT=off
  mux1 : Mux  Inputs=2
  mux2 : Mux  Inputs=2
  beta [deg] : Outport
  wires:
  Sum/1 -> Integrator/1
  fault 5/1 -> Compare To Constant/1
  Signal Specification/1 -> beta [deg]/1
  mux2/1 -> Switch1/3
  Constant1/1 -> mux1/2
  mux1/1 -> Switch1/1
  Product5/1 -> Gain2/1
  Product2/1 -> Sum/3
  Demux1/1 -> Product5/1, Square/1
  Constant2/1 -> Sum1/2
  Integrator/1 -> Product2/1, Integrator1/1
  Demux1/2 -> Product5/2
  Integrator1/1 -> Signal Specification/1, Product3/2
  Gain2/1 -> Product2/2
  Switch1/1 -> Demux1/1
  Constant3/1 -> mux2/1
  Constant/1 -> mux1/1
  Product3/1 -> Sum/1
  Product1/1 -> Sum/2
  Square/1 -> Product3/1, Product1/2
  Constant4/1 -> mux2/2
  Sum1/1 -> Switch1/2
  Compare To Constant/1 -> Sum1/1
  beta_ref [deg]/1 -> Product1/1

== matlab function libturbines/Floating NREL5MW faulty/Sensors sampling/Generator speed sensor fault ==
  settings: updateMethod=DISCRETE
  data: w_gen_real input; w_gen_prev input; GenSenFault input; drift_aux_in input; w_gen_meas output; faultOptions parameter; drift_aux_out output
function [w_gen_meas,drift_aux_out] = fcn(w_gen_real,w_gen_prev,GenSenFault,drift_aux_in,faultOptions)
%%%%%%%%%%%%%%%%%%%%%%%%%%%%%%%%%%%%%%%%%%%%%%%%%%%%%%%%%%%%%%%%%%%%%%%%%
% Generator speed sensor fault function
% Inputs:
%   - w_gen_real:   Real generator speed [rad/s]
%   - w_gen_prev:   Previous generator speed (measured) [rad/s]
%   - fault_type:   Desired fault type:
%                     0 - no fault
%                     1 - stuck at a fixed value
%                     2 - constant offset fault
%                     3 - drifting fault
%                     4 - constant gain fault
%                     5 - loss of precision
% Outputs:
%   - w_gen_meas:   Measured generator speed [rad/s] after the effect of the fault
%
%
% Author: Yerai Peña-Sanchez
%%%%%%%%%%%%%%%%%%%%%%%%%%%%%%%%%%%%%%%%%%%%%%%%%%%%%%%%%%%%%%%%%%%%%%%%

y_t = w_gen_real;  % Without any fault
switch floor(GenSenFault)
    case 1  % Stuck at a fixed value
        y_t = w_gen_prev;
    case 2  % Constant offset value
        y_t = w_gen_real-faultOptions.GenSenOffset;
    case 3  % Drifting value
        drift_aux_in = drift_aux_in + 1;
        y_t = w_gen_real + drift_aux_in*faultOptions.GenSenDriftSlope;
    case 4  % Constant gain value
        y_t = w_gen_real*faultOptions.GenSenGain;
    case 5  % Loss of precision of the sensor
        y_t = w_gen_real+w_gen_real*(2*rand-1)*faultOptions.GenSenPrecision;
end

if floor(GenSenFault) ~= 3
    drift_aux_out = 0;
else
    drift_aux_out = drift_aux_in;
end
w_gen_meas = y_t;

== matlab function libturbines/Floating IEA15MW faulty/Sensors sampling/Generator power sensor fault ==
  settings: updateMethod=DISCRETE
  data: p_gen_real input; p_gen_prev input; GenPSenFault input; drift_aux_in input; p_gen_meas output; faultOptions parameter; drift_aux_out output
function [p_gen_meas,drift_aux_out] = fcn(p_gen_real,p_gen_prev,GenPSenFault,drift_aux_in,faultOptions)
%%%%%%%%%%%%%%%%%%%%%%%%%%%%%%%%%%%%%%%%%%%%%%%%%%%%%%%%%%%%%%%%%%%%%%%%%
% Generator power sensor fault function
% Inputs:
%   - p_gen_real:   Real generator power [W]
%   - p_gen_prev:   Previous generator power (measured) [W]
%   - fault_type:   Desired fault type:
%                     0 - no fault
%                     1 - stuck at a fixed value
%                     2 - constant offset fault
%                     3 - drifting fault
%                     4 - constant gain fault
%                     5 - loss of precision
% Outputs:
%   - p_gen_meas:   Measured generator power [W] after the effect of the fault
%
%
% Author: Yerai Peña-Sanchez
%%%%%%%%%%%%%%%%%%%%%%%%%%%%%%%%%%%%%%%%%%%%%%%%%%%%%%%%%%%%%%%%%%%%%%%%

y_t = p_gen_real;  % Without any fault
switch floor(GenPSenFault)
    case 1  % Stuck at a fixed value
        y_t = p_gen_prev;
    case 2  % Constant offset value
        y_t = p_gen_real-faultOptions.GenPSenOffset;
    case 3  % Drifting value
        drift_aux_in = drift_aux_in + 1;
        y_t = p_gen_real + drift_aux_in*faultOptions.GenPSenDriftSlope;
    case 4  % Constant gain value
        y_t = p_gen_real*faultOptions.GenPSenGain;
    case 5  % Loss of precision of the sensor
        y_t = p_gen_real+p_gen_real*(2*rand-1)*faultOptions.GenPSenPrecision;
end

if floor(GenPSenFault) ~= 3
    drift_aux_out = 0;
else
    drift_aux_out = drift_aux_in;
end
p_gen_meas = y_t;

== matlab function libturbines/Floating NREL5MW faulty/Sensors sampling/Rotor speed sensor fault ==
  settings: updateMethod=DISCRETE
  data: w_rot_real input; w_rot_prev input; RotSenFault input; drift_aux_in input; w_rot_meas output; faultOptions parameter; drift_aux_out output
function [w_rot_meas,drift_aux_out] = fcn(w_rot_real,w_rot_prev,RotSenFault,drift_aux_in,faultOptions)
%%%%%%%%%%%%%%%%%%%%%%%%%%%%%%%%%%%%%%%%%%%%%%%%%%%%%%%%%%%%%%%%%%%%%%%%%
% Rotor speed sensor fault function
% Inputs:
%   - w_gen_real:   Real rotor speed [rad/s]
%   - w_gen_prev:   Previous generator speed (measured) [rad/s]
%   - fault_type:   Desired fault type:
%                     0 - no fault
%                     1 - stuck at a fixed value
%                     2 - constant offset fault
%                     3 - drifting fault
%                     4 - constant gain fault
%                     5 - loss of precision
% Outputs:
%   - w_rot_meas:   Measured rotor speed [rad/s] after the effect of the fault
%
%
% Author: Yerai Peña-Sanchez
%%%%%%%%%%%%%%%%%%%%%%%%%%%%%%%%%%%%%%%%%%%%%%%%%%%%%%%%%%%%%%%%%%%%%%%%

y_t = w_rot_real;  % Without any fault
switch floor(RotSenFault)
    case 1  % Stuck at a fixed value
        y_t = w_rot_prev;
    case 2  % Constant offset value
        y_t = w_rot_real-faultOptions.RotSenOffset;
    case 3  % Drifting value
        drift_aux_in = drift_aux_in + 1;
        y_t = w_rot_real + drift_aux_in*faultOptions.RotSenDriftSlope;
    case 4  % Constant gain value
        y_t = w_rot_real*faultOptions.RotSenGain;
    case 5  % Loss of precision of the sensor
        y_t = w_rot_real+w_rot_real*(2*rand-1)*faultOptions.RotSenPrecision;
end

if floor(RotSenFault) ~= 3
    drift_aux_out = 0;
else
    drift_aux_out = drift_aux_in;
end
w_rot_meas = y_t;

== matlab function libturbines/Floating NREL5MW faulty/Sensors sampling/Generator power sensor fault ==
  settings: updateMethod=DISCRETE
  data: p_gen_real input; p_gen_prev input; GenPSenFault input; drift_aux_in input; p_gen_meas output; faultOptions parameter; drift_aux_out output
function [p_gen_meas,drift_aux_out] = fcn(p_gen_real,p_gen_prev,GenPSenFault,drift_aux_in,faultOptions)
%%%%%%%%%%%%%%%%%%%%%%%%%%%%%%%%%%%%%%%%%%%%%%%%%%%%%%%%%%%%%%%%%%%%%%%%%
% Generator power sensor fault function
% Inputs:
%   - p_gen_real:   Real generator power [W]
%   - p_gen_prev:   Previous generator power (measured) [W]
%   - fault_type:   Desired fault type:
%                     0 - no fault
%                     1 - stuck at a fixed value
%                     2 - constant offset fault
%                     3 - drifting fault
%                     4 - constant gain fault
%                     5 - loss of precision
% Outputs:
%   - p_gen_meas:   Measured generator power [W] after the effect of the fault
%
%
% Author: Yerai Peña-Sanchez
%%%%%%%%%%%%%%%%%%%%%%%%%%%%%%%%%%%%%%%%%%%%%%%%%%%%%%%%%%%%%%%%%%%%%%%%

y_t = p_gen_real;  % Without any fault
switch floor(GenPSenFault)
    case 1  % Stuck at a fixed value
        y_t = p_gen_prev;
    case 2  % Constant offset value
        y_t = p_gen_real-faultOptions.GenPSenOffset;
    case 3  % Drifting value
        drift_aux_in = drift_aux_in + 1;
        y_t = p_gen_real + drift_aux_in*faultOptions.GenPSenDriftSlope;
    case 4  % Constant gain value
        y_t = p_gen_real*faultOptions.GenPSenGain;
    case 5  % Loss of precision of the sensor
        y_t = p_gen_real+p_gen_real*(2*rand-1)*faultOptions.GenPSenPrecision;
end

if floor(GenPSenFault) ~= 3
    drift_aux_out = 0;
else
    drift_aux_out = drift_aux_in;
end
p_gen_meas = y_t;

== matlab function libturbines/Floating IEA15MW faulty/Sensors sampling/Generator speed sensor fault ==
  settings: updateMethod=DISCRETE
  data: w_gen_real input; w_gen_prev input; GenSenFault input; drift_aux_in input; w_gen_meas output; faultOptions parameter; drift_aux_out output
function [w_gen_meas,drift_aux_out] = fcn(w_gen_real,w_gen_prev,GenSenFault,drift_aux_in,faultOptions)
%%%%%%%%%%%%%%%%%%%%%%%%%%%%%%%%%%%%%%%%%%%%%%%%%%%%%%%%%%%%%%%%%%%%%%%%%
% Generator speed sensor fault function
% Inputs:
%   - w_gen_real:   Real generator speed [rad/s]
%   - w_gen_prev:   Previous generator speed (measured) [rad/s]
%   - fault_type:   Desired fault type:
%                     0 - no fault
%                     1 - stuck at a fixed value
%                     2 - constant offset fault
%                     3 - drifting fault
%                     4 - constant gain fault
%                     5 - loss of precision
% Outputs:
%   - w_gen_meas:   Measured generator speed [rad/s] after the effect of the fault
%
%
% Author: Yerai Peña-Sanchez
%%%%%%%%%%%%%%%%%%%%%%%%%%%%%%%%%%%%%%%%%%%%%%%%%%%%%%%%%%%%%%%%%%%%%%%%

y_t = w_gen_real;  % Without any fault
switch floor(GenSenFault)
    case 1  % Stuck at a fixed value
        y_t = w_gen_prev;
    case 2  % Constant offset value
        y_t = w_gen_real-faultOptions.GenSenOffset;
    case 3  % Drifting value
        drift_aux_in = drift_aux_in + 1;
        y_t = w_gen_real + drift_aux_in*faultOptions.GenSenDriftSlope;
    case 4  % Constant gain value
        y_t = w_gen_real*faultOptions.GenSenGain;
    case 5  % Loss of precision of the sensor
        y_t = w_gen_real+w_gen_real*(2*rand-1)*faultOptions.GenSenPrecision;
end

if floor(GenSenFault) ~= 3
    drift_aux_out = 0;
else
    drift_aux_out = drift_aux_in;
end
w_gen_meas = y_t;

== matlab function libturbines/Floating IEA15MW faulty/Sensors sampling/Pitch sensor fault ==
  settings: updateMethod=DISCRETE
  data: beta_real input; beta_prev input; PitchSenFault input; drift_aux_in input; beta_meas output; faultOptions parameter; drift_aux_out output
function [beta_meas,drift_aux_out] = fcn(beta_real,beta_prev,PitchSenFault,drift_aux_in,faultOptions)
%%%%%%%%%%%%%%%%%%%%%%%%%%%%%%%%%%%%%%%%%%%%%%%%%%%%%%%%%%%%%%%%%%%%%%%%%
% Pitch sensor fault function
% Inputs:
%   - beta_real:    Real pitch angle [deg] of the actuator
%   - beta_prev:    Previous pitch angle (measured) [deg]
%   - fault_type:   Desired fault type:
%                     0 - no fault
%                     1 - stuck at a fixed value
%                     2 - constant offset fault
%                     3 - drifting fault
%                     4 - constant gain fault
%                     5 - loss of precision
% Outputs:
%   - beta_meas:    Measured pitch angle [deg] after the effect of the fault
%
%
% Author: Yerai Peña-Sanchez
%%%%%%%%%%%%%%%%%%%%%%%%%%%%%%%%%%%%%%%%%%%%%%%%%%%%%%%%%%%%%%%%%%%%%%%%

y_t = beta_real;  % Without any fault
switch floor(PitchSenFault)
    case 1  % Stuck at a fixed value
        y_t(3) = beta_prev(3);
    case 2  % Constant offset value
        y_t(3) = beta_real(3)-faultOptions.PitchSenOffset;
    case 3  % Drifting value
        drift_aux_in = drift_aux_in + 1;
        y_t(3) = beta_real(3) + drift_aux_in*faultOptions.PitchSenDriftSlope;
    case 4  % Constant gain value
        y_t(3) = beta_real(3)*faultOptions.PitchSenGain;
    case 5  % Loss of precision of the sensor
        y_t(3) = beta_real(3)+beta_real(3)*(2*rand-1)*faultOptions.PitchSenPrecision;
end

if floor(PitchSenFault) ~= 3
    drift_aux_out = 0;
else
    drift_aux_out = drift_aux_in;
end
% beta_meas = [y_t; beta_real; beta_real];
beta_meas = y_t;

== matlab function libturbines/Floating IEA15MW faulty/Sensors sampling/Rotor speed sensor fault ==
  settings: updateMethod=DISCRETE
  data: w_rot_real input; w_rot_prev input; RotSenFault input; drift_aux_in input; w_rot_meas output; faultOptions parameter; drift_aux_out output
function [w_rot_meas,drift_aux_out] = fcn(w_rot_real,w_rot_prev,RotSenFault,drift_aux_in,faultOptions)
%%%%%%%%%%%%%%%%%%%%%%%%%%%%%%%%%%%%%%%%%%%%%%%%%%%%%%%%%%%%%%%%%%%%%%%%%
% Rotor speed sensor fault function
% Inputs:
%   - w_gen_real:   Real rotor speed [rad/s]
%   - w_gen_prev:   Previous generator speed (measured) [rad/s]
%   - fault_type:   Desired fault type:
%                     0 - no fault
%                     1 - stuck at a fixed value
%                     2 - constant offset fault
%                     3 - drifting fault
%                     4 - constant gain fault
%                     5 - loss of precision
% Outputs:
%   - w_rot_meas:   Measured rotor speed [rad/s] after the effect of the fault
%
%
% Author: Yerai Peña-Sanchez
%%%%%%%%%%%%%%%%%%%%%%%%%%%%%%%%%%%%%%%%%%%%%%%%%%%%%%%%%%%%%%%%%%%%%%%%

y_t = w_rot_real;  % Without any fault
switch floor(RotSenFault)
    case 1  % Stuck at a fixed value
        y_t = w_rot_prev;
    case 2  % Constant offset value
        y_t = w_rot_real-faultOptions.RotSenOffset;
    case 3  % Drifting value
        drift_aux_in = drift_aux_in + 1;
        y_t = w_rot_real + drift_aux_in*faultOptions.RotSenDriftSlope;
    case 4  % Constant gain value
        y_t = w_rot_real*faultOptions.RotSenGain;
    case 5  % Loss of precision of the sensor
        y_t = w_rot_real+w_rot_real*(2*rand-1)*faultOptions.RotSenPrecision;
end

if floor(RotSenFault) ~= 3
    drift_aux_out = 0;
else
    drift_aux_out = drift_aux_in;
end
w_rot_meas = y_t;

== matlab function libturbines/Floating IEA3.4MW faulty/Generator simple/Generator fault ==
  data: GenActFault input; torque input; torque_prev input; drift_aux_in input; torque_real output; faultOptions parameter; drift_aux_out output
function [torque_real,drift_aux_out] = fcn(GenActFault,torque,torque_prev,drift_aux_in,faultOptions)
%%%%%%%%%%%%%%%%%%%%%%%%%%%%%%%%%%%%%%%%%%%%%%%%%%%%%%%%%%%%%%%%%%%%%%%%%
% Generator fault function
% Inputs:
%   - torque:       Reference torque value [Nm] from the controller
%   - fault_type:   Desired fault type:
%                     0 - no fault
%                     1 - stuck at a fixed value
%                     2 - constant offset fault
%                     3 - loss of efectiveness (in a different function)
% Outputs:
%   - torque_real:  Real torque value [Nm] after the effect of the fault
%
%
% Author: Yerai Peña-Sanchez
%%%%%%%%%%%%%%%%%%%%%%%%%%%%%%%%%%%%%%%%%%%%%%%%%%%%%%%%%%%%%%%%%%%%%%%%

y_t = torque;  % Without any fault
switch floor(GenActFault)
    case 1  % Stuck generator
        y_t = torque_prev;
    case 2  % Constant offset value
        y_t = y_t-faultOptions.GenActOffset;
    case 3  % Drifting value
        drift_aux_in = drift_aux_in + 1;
        y_t = y_t + drift_aux_in*faultOptions.GenActDriftSlope;
    case 4  % Constant gain value
        y_t = y_t*faultOptions.GenActGain;
end

if floor(GenActFault) ~= 3
    drift_aux_out = 0;
else
    drift_aux_out = drift_aux_in;
end

torque_real = y_t;

== matlab function libturbines/Floating IEA3.4MW faulty/Generator simple/Generator fault type 3 ==
  data: GenActFault input; out output; faultOptions parameter
function out = fcn(GenActFault,faultOptions)
%%%%%%%%%%%%%%%%%%%%%%%%%%%%%%%%%%%%%%%%%%%%%%%%%%%%%%%%%%%%%%%%%%%%%%%%%
% Generator loss of effectiveness fault type signal generator
% Inputs:
%   - fault_type:   Desired fault type:
%                     0 - no fault
%                     1 - stuck at a fixed value (in a different function)
%                     2 - constant offset fault (in a different function)
%                     3 - loss of efectiveness
% Outputs:
%   - out:          Signal for the loss of effectiveness fault and the faulty signal
%
%
% Author: Yerai Peña-Sanchez
%%%%%%%%%%%%%%%%%%%%%%%%%%%%%%%%%%%%%%%%%%%%%%%%%%%%%%%%%%%%%%%%%%%%%%%%

out = [GenActFault ; 1];              % Without any fault
if GenActFault == 3                   % Loss of effectiveness fault
    out(2) = faultOptions.GenActEffectiveness;
end
